simulink model "sensorMCUSlugsMKII_greg"  (Simulink 6.6)
settings: Solver=FixedStepDiscrete  StartTime=0.0  StopTime=10.0  FixedStep=0.01  RelTol=1e-3
InitFcn:
  | mcuInit
values from neighbouring files (symbols this model uses):
  T = 0.01    [initGPS.m]    (also in mcuInit.m)
undefined symbols (not defined in the file or in its folder): baroMeanTemp, baroOffset, baroScale, baroTempK, baseHeight, baseTemp, cubeAccelGain, cubeGyroGain, gaind, getCubeData, getGpsMainData, getMag, hil_getEuler, hil_getRates, hil_getRawRead, hil_getVned, hil_getXYZ, hilRead, ISA_rho0, lapseRate, logData, magMeanTemp, magOffset, magScale, magTempK, pitMeanTemp, pitotOffset, pitotScale, pitTempK, polesd, powerOffset, powerScale, protParseDecode, sensorMCUInit, spiSend, tempOffset, tempScale, u1, u2, updateAirData, updateAttitude, updateBias, updateDiagnosticFl, updateDiagnosticSh, updateLoadData, updatePilotConsole, updatePosition, updateRawADCData, updateTimeStamp, y1, zerosd
libraries: dsPICdrivers x36, simulink x3, aerolibconvert2 x1
(part 2 of 2)

== system sensorMCUSlugsMKII_greg/Sensor Data/Sensor Suite/Low Pass Filtering,Temperature Compensation and Calibration/3D Filter ==
  In1 : Inport
  Demux : Demux  Outputs=3
  Filter1 : Subsystem  mask(DiscretizedZeroPole){Zeros=zval, Poles=pval, Gain=kval, AbsTol=auto, SampleTime=TSample, method=tustin, Wc=1}
      mask prompts: Zeros "Zeros (enter in s-main:)"; Poles "Poles (enter in s-domain:)"; Gain "Gain (enter in s-domain:)"; AbsTol "Absolute tolerance:"; SampleTime "Sample time:"; Wc "Critical Frequency (Hz):"
      mask help: Continuous mask uses c2d to transform parameters onto the Discrete Zero-Pole block inside.
      mask init: same as sensorMCUSlugsMKII_greg/Sensor Data/Sensor Suite/Low Pass Filtering,Temperature Compensation and Calibration/Low Pass1
      mask StyleString: edit,edit,edit,edit,edit,popup(zoh|foh|tustin|prewarp|matched),edit
      mask CallbackString: |||||hidecrit|
      mask Display:
      | droots(zeross,poless,gainss)
      | text( 0.5, 1.0, method, 'verticalAlignment','top')
  Filter2 : Subsystem  mask(DiscretizedZeroPole){Zeros=zval, Poles=pval, Gain=kval, AbsTol=auto, SampleTime=TSample, method=tustin, Wc=1}
      mask prompts: Zeros "Zeros (enter in s-main:)"; Poles "Poles (enter in s-domain:)"; Gain "Gain (enter in s-domain:)"; AbsTol "Absolute tolerance:"; SampleTime "Sample time:"; Wc "Critical Frequency (Hz):"
      mask help: Continuous mask uses c2d to transform parameters onto the Discrete Zero-Pole block inside.
      mask init: same as sensorMCUSlugsMKII_greg/Sensor Data/Sensor Suite/Low Pass Filtering,Temperature Compensation and Calibration/Low Pass1
      mask StyleString: edit,edit,edit,edit,edit,popup(zoh|foh|tustin|prewarp|matched),edit
      mask CallbackString: |||||hidecrit|
      mask Display:
      | droots(zeross,poless,gainss)
      | text( 0.5, 1.0, method, 'verticalAlignment','top')
  Filter3 : Subsystem  mask(DiscretizedZeroPole){Zeros=zval, Poles=pval, Gain=kval, AbsTol=auto, SampleTime=TSample, method=tustin, Wc=1}
      mask prompts: Zeros "Zeros (enter in s-main:)"; Poles "Poles (enter in s-domain:)"; Gain "Gain (enter in s-domain:)"; AbsTol "Absolute tolerance:"; SampleTime "Sample time:"; Wc "Critical Frequency (Hz):"
      mask help: Continuous mask uses c2d to transform parameters onto the Discrete Zero-Pole block inside.
      mask init: same as sensorMCUSlugsMKII_greg/Sensor Data/Sensor Suite/Low Pass Filtering,Temperature Compensation and Calibration/Low Pass1
      mask StyleString: edit,edit,edit,edit,edit,popup(zoh|foh|tustin|prewarp|matched),edit
      mask CallbackString: |||||hidecrit|
      mask Display:
      | droots(zeross,poless,gainss)
      | text( 0.5, 1.0, method, 'verticalAlignment','top')
  myMux Fun1 : Stateflow chart
  Out1 : Outport
  wires:
  myMux Fun1/1(y) -> Out1/1
  In1/1 -> Demux/1
  Filter3/1(Out1) -> myMux Fun1/3(u3)
  Filter2/1(Out1) -> myMux Fun1/2(u2)
  Filter1/1(Out1) -> myMux Fun1/1(u1)
  Demux/3 -> Filter3/1(In1)
  Demux/2 -> Filter2/1(In1)
  Demux/1 -> Filter1/1(In1)

== system sensorMCUSlugsMKII_greg/Sensor Data/Sensor Suite/Low Pass Filtering,Temperature Compensation and Calibration/Baro Altimeter ==
  Static (Pa) : Inport  Orientation=up
  Compute Barometric Height : Subsystem  mask{baseTemp=baseTemp, LapseRate=lapseRate}
      mask prompts: baseTemp "Base Station Temperature (K)"; LapseRate "Lapse Rate (C/ft)"
      mask help:
      | Produces Altitude in meters from Barometric Pressure in Pascals. Altitude is valid from MSL to 6000 ft.
      |
      | The method implemented here was developed by Ren Curry
  Constant1 : Constant  Value=baseHeight  OutDataTypeMode=single
  Enabled Subsystem : Subsystem  TreatAsAtomicUnit=on
  Enables/Disables the Computation of  initial Baro Bias : Stateflow chart
  Initial Baro Bias : Subsystem  TreatAsAtomicUnit=on
  Logical Operator : Logic  Orientation=down  Operator=NOT  AllPortsSameDT=off  OutDataTypeMode=Boolean
  Sum1 : Sum  Inputs=++|  OutDataTypeMode=single
  Zero Out Height : Subsystem  TreatAsAtomicUnit=on
  Altitude : Outport
  wires:
  Compute Barometric Height/1("Altitude, m") -> Zero Out Height/2(Computed Height), Sum1/2
  Static (Pa)/1 -> Initial Baro Bias/1(Baro (Pa)), Compute Barometric Height/3(Baro (Pa))
  Enables/Disables the Computation of  initial Baro Bias/1(tOut) -> Initial Baro Bias/Enable, Zero Out Height/Enable, Logical Operator/1
  Constant1/1 -> Compute Barometric Height/1(Base Height (m)), Zero Out Height/1(Base Height)
  Initial Baro Bias/1(Baro (Gnd)) -> Compute Barometric Height/2(Base Pressure (Pa))
  Zero Out Height/1(Height Offset) -> Sum1/1
  Logical Operator/1 -> Enabled Subsystem/Enable
  Sum1/1 -> Enabled Subsystem/1(In1)
  Enabled Subsystem/1(Out1) -> Altitude/1

== system sensorMCUSlugsMKII_greg/Sensor Data/Sensor Suite/Low Pass Filtering,Temperature Compensation and Calibration/Baro Temp Compensation ==
  Raw : Inport
  Temp Raw : Inport  Port=2
  Divide1 : Product  OutDataTypeMode=single  OutScaling=2^-10
  Mean Temperature for Calibration : Constant  Value=tempMean  OutDataTypeMode=single
  Sum1 : Sum  Inputs=|+-  OutDataTypeMode=single
  Sum2 : Sum  Inputs=|+-  OutDataTypeMode=single
  gains : Constant  Value=alpha  OutDataTypeMode=single
  Comp : Outport
  wires:
  Mean Temperature for Calibration/1 -> Sum1/2
  Raw/1 -> Sum2/1
  Temp Raw/1 -> Sum1/1
  Sum1/1 -> Divide1/2
  gains/1 -> Divide1/1
  Divide1/1 -> Sum2/2
  Sum2/1 -> Comp/1

== system sensorMCUSlugsMKII_greg/Sensor Data/Sensor Suite/Low Pass Filtering,Temperature Compensation and Calibration/Barometer Unit Conversion ==
  Raw : Inport
  Bias : Constant  Value=bias  OutDataTypeMode=single
  Divide : Product  OutDataTypeMode=single  OutScaling=2^-10
  Gains : Constant  Value=gains  OutDataTypeMode=single
  Sum : Sum  Inputs=|++  OutDataTypeMode=single
  Comp : Outport
  wires:
  Bias/1 -> Sum/2
  Raw/1 -> Divide/2
  Gains/1 -> Divide/1
  Divide/1 -> Sum/1
  Sum/1 -> Comp/1

== system sensorMCUSlugsMKII_greg/Sensor Data/Sensor Suite/Low Pass Filtering,Temperature Compensation and Calibration/Low Pass1 ==
  In1 : Inport
  Discrete Zero-Pole : DiscreteZeroPole  Zeros=zerosd  Poles=polesd  Gain=gaind  SampleTime=SampleTime
  Out1 : Outport
  wires:
  In1/1 -> Discrete Zero-Pole/1
  Discrete Zero-Pole/1 -> Out1/1

== system sensorMCUSlugsMKII_greg/Sensor Data/Sensor Suite/Low Pass Filtering,Temperature Compensation and Calibration/Low Pass2 ==
  In1 : Inport
  Discrete Zero-Pole : DiscreteZeroPole  Zeros=zerosd  Poles=polesd  Gain=gaind  SampleTime=SampleTime
  Out1 : Outport
  wires:
  Discrete Zero-Pole/1 -> Out1/1
  In1/1 -> Discrete Zero-Pole/1

== system sensorMCUSlugsMKII_greg/Sensor Data/Sensor Suite/Low Pass Filtering,Temperature Compensation and Calibration/Low Pass4 ==
  In1 : Inport
  Discrete Zero-Pole : DiscreteZeroPole  Zeros=zerosd  Poles=polesd  Gain=gaind  SampleTime=SampleTime
  Out1 : Outport
  wires:
  Discrete Zero-Pole/1 -> Out1/1
  In1/1 -> Discrete Zero-Pole/1

== system sensorMCUSlugsMKII_greg/Sensor Data/Sensor Suite/Low Pass Filtering,Temperature Compensation and Calibration/Low Pass8 ==
  In1 : Inport
  Discrete Zero-Pole : DiscreteZeroPole  Zeros=zerosd  Poles=polesd  Gain=gaind  SampleTime=SampleTime
  Out1 : Outport
  wires:
  In1/1 -> Discrete Zero-Pole/1
  Discrete Zero-Pole/1 -> Out1/1

== system sensorMCUSlugsMKII_greg/Sensor Data/Sensor Suite/Low Pass Filtering,Temperature Compensation and Calibration/Magnetometer Unit Conversion ==
  Raw : Inport
  Bias : Constant  Value=bias  OutDataTypeMode=single
  Divide : Product  OutDataTypeMode=single  OutScaling=2^-10
  Gains : Constant  Value=gains  OutDataTypeMode=single
  Sum : Sum  Inputs=|++  OutDataTypeMode=single
  Comp : Outport
  wires:
  Sum/1 -> Comp/1
  Divide/1 -> Sum/1
  Gains/1 -> Divide/1
  Raw/1 -> Divide/2
  Bias/1 -> Sum/2

== system sensorMCUSlugsMKII_greg/Sensor Data/Sensor Suite/Low Pass Filtering,Temperature Compensation and Calibration/Magnetometers Temp Compensation ==
  Raw : Inport
  Temp Raw : Inport  Port=2
  Divide1 : Product  OutDataTypeMode=single  OutScaling=2^-10
  Mean Temperature for Calibration : Constant  Value=tempMean  OutDataTypeMode=single
  Sum1 : Sum  Inputs=|+-  OutDataTypeMode=single
  Sum2 : Sum  Inputs=|+-  OutDataTypeMode=single
  gains : Constant  Value=alpha  OutDataTypeMode=single
  Comp : Outport
  wires:
  Sum2/1 -> Comp/1
  Divide1/1 -> Sum2/2
  gains/1 -> Divide1/1
  Sum1/1 -> Divide1/2
  Temp Raw/1 -> Sum1/1
  Raw/1 -> Sum2/1
  Mean Temperature for Calibration/1 -> Sum1/2

== system sensorMCUSlugsMKII_greg/Sensor Data/Sensor Suite/Low Pass Filtering,Temperature Compensation and Calibration/Pitot Unit Conversion ==
  Raw : Inport
  Bias : Constant  Value=bias  OutDataTypeMode=single
  Divide : Product  OutDataTypeMode=single  OutScaling=2^-10
  Gains : Constant  Value=gains  OutDataTypeMode=single
  Sum : Sum  Inputs=|++  OutDataTypeMode=single
  Comp : Outport
  wires:
  Bias/1 -> Sum/2
  Raw/1 -> Divide/2
  Gains/1 -> Divide/1
  Divide/1 -> Sum/1
  Sum/1 -> Comp/1

== system sensorMCUSlugsMKII_greg/Sensor Data/Sensor Suite/Low Pass Filtering,Temperature Compensation and Calibration/Pitot Temp Compensation ==
  Raw : Inport
  Temp Raw : Inport  Port=2
  Divide1 : Product  OutDataTypeMode=single  OutScaling=2^-10
  Mean Temperature for Calibration : Constant  Value=tempMean  OutDataTypeMode=single
  Sum1 : Sum  Inputs=|+-  OutDataTypeMode=single
  Sum2 : Sum  Inputs=|+-  OutDataTypeMode=single
  gains : Constant  Value=alpha  OutDataTypeMode=single
  Comp : Outport
  wires:
  Mean Temperature for Calibration/1 -> Sum1/2
  Raw/1 -> Sum2/1
  Temp Raw/1 -> Sum1/1
  Sum1/1 -> Divide1/2
  gains/1 -> Divide1/1
  Divide1/1 -> Sum2/2
  Sum2/1 -> Comp/1

== system sensorMCUSlugsMKII_greg/Sensor Data/Sensor Suite/Low Pass Filtering,Temperature Compensation and Calibration/Power Unit Conversion ==
  Raw : Inport
  Bias : Constant  Value=bias  OutDataTypeMode=single
  Divide : Product  OutDataTypeMode=single  OutScaling=2^-10
  Gains : Constant  Value=gains  OutDataTypeMode=single
  Sum : Sum  Inputs=|++  OutDataTypeMode=single
  Comp : Outport
  wires:
  Bias/1 -> Sum/2
  Raw/1 -> Divide/2
  Gains/1 -> Divide/1
  Divide/1 -> Sum/1
  Sum/1 -> Comp/1

== system sensorMCUSlugsMKII_greg/Sensor Data/Sensor Suite/Low Pass Filtering,Temperature Compensation and Calibration/Thermistor Unit Conversion ==
  Raw : Inport
  Bias : Constant  Value=bias  OutDataTypeMode=single
  Divide : Product  OutDataTypeMode=single  OutScaling=2^-10
  Gains : Constant  Value=gains  OutDataTypeMode=single
  Sum : Sum  Inputs=|++  OutDataTypeMode=single
  Comp : Outport
  wires:
  Sum/1 -> Comp/1
  Divide/1 -> Sum/1
  Gains/1 -> Divide/1
  Raw/1 -> Divide/2
  Bias/1 -> Sum/2

== system sensorMCUSlugsMKII_greg/Position-Attitude Filter/Position Filter/Geod2LTP2/ECEF2LTP (UEN)/From Body to Universal1 ==
  long : Inport
  lat : Inport  Port=2
  Mux : Mux  Inputs=2
  Reshape 9x1->3x1 : S-Function  FunctionName=sreshape  Parameters=OutputDimensionality, OutputDimensions  mask(Reshape){OutputDimensionality=Customize, OutputDimensions=[3,3]}
      mask prompts: OutputDimensionality "Output dimensionality:"; OutputDimensions "Output dimensions:"
      mask help:
      | Change the dimensions of a vector or matrix input signal. Output
      |  - a one-dimensional array (vector),
      |  - a column vector (Mx1 matrix),
      |  - a row vector (1xN matrix), or
      |  - a matrix or vector with specified dimensions, e.g., [M, N] or [W].
      mask init:
      | s = reshapemask(gcb,'init');
      mask StyleString: popup(1-D array|Column vector|Row vector|Customize),edit
      mask CallbackString: reshapemask(gcb,'cbDimensionality')|
      mask Display: disp('Reshape')
  Rotation Matrix from Long//Lat : Subsystem
      mask Type: Vector Transformation
      mask Description: Vector Transformation
      mask Display: disp('axis')
  DCM : Outport
  wires:
  lat/1 -> Mux/2
  long/1 -> Mux/1
  Mux/1 -> Rotation Matrix from Long//Lat/1(long lat)
  Rotation Matrix from Long//Lat/1(DCM) -> Reshape 9x1->3x1/1
  Reshape 9x1->3x1/1 -> DCM/1

== system sensorMCUSlugsMKII_greg/Position-Attitude Filter/Position Filter/Geod2LTP2/Geod2ECEF/eccentricity^2 ==
  " " : Product  SaturateOnIntegerOverflow=on  InputSameDT=on
  Re=equatorial radius1 : Constant  Value=Re
  Rp=polar radius : Constant  Value=Rp
  Sum5 : Sum  Inputs=|+-  SaturateOnIntegerOverflow=on  InputSameDT=on
  const2 : Constant
  e^1 : Product  Inputs=*/  SaturateOnIntegerOverflow=on  InputSameDT=on
  e^2 : Outport
  wires:
  Re=equatorial radius1/1 -> e^1/2
  Rp=polar radius/1 -> e^1/1
  const2/1 -> Sum5/1
  e^1/1 -> " "/2, " "/1
  " "/1 -> Sum5/2
  Sum5/1 -> e^2/1

== system sensorMCUSlugsMKII_greg/Position-Attitude Filter/Position Filter/Geod2LTP2/Geod2ECEF1/eccentricity^2 ==
  " " : Product  SaturateOnIntegerOverflow=on  InputSameDT=on
  Re=equatorial radius1 : Constant  Value=Re
  Rp=polar radius : Constant  Value=Rp
  Sum5 : Sum  Inputs=|+-  SaturateOnIntegerOverflow=on  InputSameDT=on
  const2 : Constant
  e^1 : Product  Inputs=*/  SaturateOnIntegerOverflow=on  InputSameDT=on
  e^2 : Outport
  wires:
  Sum5/1 -> e^2/1
  " "/1 -> Sum5/2
  e^1/1 -> " "/1, " "/2
  const2/1 -> Sum5/1
  Rp=polar radius/1 -> e^1/1
  Re=equatorial radius1/1 -> e^1/2

== system sensorMCUSlugsMKII_greg/Sensor Data/Sensor Suite/Low Pass Filtering,Temperature Compensation and Calibration/3D Filter/Filter1 ==
  In1 : Inport
  Discrete Zero-Pole : DiscreteZeroPole  Zeros=zerosd  Poles=polesd  Gain=gaind  SampleTime=SampleTime
  Out1 : Outport
  wires:
  Discrete Zero-Pole/1 -> Out1/1
  In1/1 -> Discrete Zero-Pole/1

== system sensorMCUSlugsMKII_greg/Sensor Data/Sensor Suite/Low Pass Filtering,Temperature Compensation and Calibration/3D Filter/Filter2 ==
  In1 : Inport
  Discrete Zero-Pole : DiscreteZeroPole  Zeros=zerosd  Poles=polesd  Gain=gaind  SampleTime=SampleTime
  Out1 : Outport
  wires:
  In1/1 -> Discrete Zero-Pole/1
  Discrete Zero-Pole/1 -> Out1/1

== system sensorMCUSlugsMKII_greg/Sensor Data/Sensor Suite/Low Pass Filtering,Temperature Compensation and Calibration/3D Filter/Filter3 ==
  In1 : Inport
  Discrete Zero-Pole : DiscreteZeroPole  Zeros=zerosd  Poles=polesd  Gain=gaind  SampleTime=SampleTime
  Out1 : Outport
  wires:
  Discrete Zero-Pole/1 -> Out1/1
  In1/1 -> Discrete Zero-Pole/1

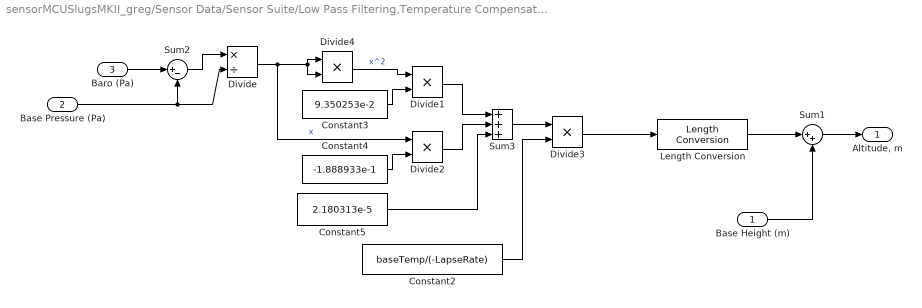
== system sensorMCUSlugsMKII_greg/Sensor Data/Sensor Suite/Low Pass Filtering,Temperature Compensation and Calibration/Baro Altimeter/Compute Barometric Height ==
  Base Height (m) : Inport
  Base Pressure (Pa) : Inport  Port=2
  Baro (Pa) : Inport  Port=3
  Constant2 : Constant  Value=baseTemp/(-LapseRate)  OutDataTypeMode=single
  Constant3 : Constant  Value=9.350253e-2  OutDataTypeMode=single
  Constant4 : Constant  Value=-1.888933e-1  OutDataTypeMode=single
  Constant5 : Constant  Value=2.180313e-5  OutDataTypeMode=single
  Divide : Product  Inputs=*/  OutDataTypeMode=single  OutScaling=2^-10
  Divide{1..4} (4 alike) : Product  OutDataTypeMode=single  OutScaling=2^-10
  Length Conversion : aerolibconvert2/Length Conversion  SystemSampleTime=-1  IU=ft  OU=m
  Sum1 : Sum  Inputs=|++  OutDataTypeMode=single
  Sum2 : Sum  Inputs=|+-  OutDataTypeMode=single
  Sum3 : Sum  Inputs=3  OutDataTypeMode=single
  "Altitude, m" : Outport
  wires:
  Length Conversion/1 -> Sum1/1
  Sum2/1 -> Divide/1
  Sum1/1 -> "Altitude, m"/1
  Divide3/1 -> Length Conversion/1
  Constant2/1 -> Divide3/2
  Sum3/1 -> Divide3/1
  Constant5/1 -> Sum3/3
  Divide2/1 -> Sum3/2
  Divide1/1 -> Sum3/1
  Constant4/1 -> Divide2/2
  Constant3/1 -> Divide1/2
  Divide4/1 -> Divide1/1  "x^2"
  Divide/1 -> Divide2/1, Divide4/1, Divide4/2  "x"
  Base Pressure (Pa)/1 -> Divide/2, Sum2/2
  Base Height (m)/1 -> Sum1/2
  Baro (Pa)/1 -> Sum2/1

== system sensorMCUSlugsMKII_greg/Sensor Data/Sensor Suite/Low Pass Filtering,Temperature Compensation and Calibration/Baro Altimeter/Enabled Subsystem ==
  In1 : Inport
  Enable : EnablePort
  Out1 : Outport  InitialOutput=baseHeight
  wires:
  In1/1 -> Out1/1

== system sensorMCUSlugsMKII_greg/Sensor Data/Sensor Suite/Low Pass Filtering,Temperature Compensation and Calibration/Baro Altimeter/Initial Baro Bias ==
  Baro (Pa) : Inport
  Enable : EnablePort
  Data Type Conversion : DataTypeConversion  OutDataTypeMode=double
  Data Type Conversion1 : DataTypeConversion  OutDataTypeMode=single
  Low Pass8 : Subsystem  mask(DiscretizedZeroPole){Zeros=[], Poles=[-3], Gain=3, AbsTol=auto, SampleTime=.01, method=tustin, Wc=1}
      mask prompts: Zeros "Zeros (enter in s-main:)"; Poles "Poles (enter in s-domain:)"; Gain "Gain (enter in s-domain:)"; AbsTol "Absolute tolerance:"; SampleTime "Sample time:"; Wc "Critical Frequency (Hz):"
      mask help: Continuous mask uses c2d to transform parameters onto the Discrete Zero-Pole block inside.
      mask init: same as sensorMCUSlugsMKII_greg/Sensor Data/Sensor Suite/Low Pass Filtering,Temperature Compensation and Calibration/Low Pass1
      mask StyleString: edit,edit,edit,edit,edit,popup(zoh|foh|tustin|prewarp|matched),edit
      mask CallbackString: |||||hidecrit|
      mask Display:
      | droots(zeross,poless,gainss)
      | text( 0.5, 1.0, method, 'verticalAlignment','top')
  Mux : Mux  Inputs=2
  Scope : Scope
      settings: SaveName=ScopeData8
  "[80k - 120k]" : Saturate  UpperLimit=120000  LowerLimit=80000
  Baro (Gnd) : Outport
  wires:
  Baro (Pa)/1 -> Data Type Conversion/1
  Low Pass8/1(Out1) -> Data Type Conversion1/1
  Data Type Conversion/1 -> Low Pass8/1(In1)
  Data Type Conversion1/1 -> Mux/2, "[80k - 120k]"/1
  Mux/1 -> Scope/1
  "[80k - 120k]"/1 -> Baro (Gnd)/1, Mux/1

== system sensorMCUSlugsMKII_greg/Sensor Data/Sensor Suite/Low Pass Filtering,Temperature Compensation and Calibration/Baro Altimeter/Zero Out Height ==
  Base Height : Inport
  Computed Height : Inport  Port=2
  Enable : EnablePort
  Integer Delay : simulink/Discrete/Integer Delay  vinit=0  samptime=.01  NumDelays=1
  Sum : Sum  Inputs=|+-  OutDataTypeMode=single
  Height Offset : Outport
  wires:
  Computed Height/1 -> Integer Delay/1
  Sum/1 -> Height Offset/1
  Integer Delay/1 -> Sum/2
  Base Height/1 -> Sum/1

== system sensorMCUSlugsMKII_greg/Position-Attitude Filter/Position Filter/Geod2LTP2/ECEF2LTP (UEN)/From Body to Universal1/Rotation Matrix from Long//Lat ==
  note: Calculate Coefficients of DCM Row-Wise
  long lat : Inport
  11 : Fcn  Expr=cos(u[1])*cos(u[2])
  12 : Fcn  Expr=sin(u[1])*cos(u[2])
  13 : Fcn  Expr=sin(u[2])
  21 : Fcn  Expr=-sin(u[1])
  22 : Fcn  Expr=cos(u[1])
  23 : Fcn  Expr=0
  31 : Fcn  Expr=-sin(u[2])*cos(u[1])
  32 : Fcn  Expr=-sin(u[1])*sin(u[2])
  33 : Fcn  Expr=cos(u[2])
  Mux2 : Mux  Inputs=9
  DCM : Outport  InitialOutput=0
  wires:
  33/1 -> Mux2/9
  23/1 -> Mux2/8
  13/1 -> Mux2/7
  32/1 -> Mux2/6
  22/1 -> Mux2/5
  12/1 -> Mux2/4
  31/1 -> Mux2/3
  21/1 -> Mux2/2
  11/1 -> Mux2/1
  Mux2/1 -> DCM/1
  long lat/1 -> 11/1, 33/1, 23/1, 13/1, 32/1, 22/1, 12/1, 31/1, 21/1

== system sensorMCUSlugsMKII_greg/Sensor Data/Sensor Suite/Low Pass Filtering,Temperature Compensation and Calibration/Baro Altimeter/Initial Baro Bias/Low Pass8 ==
  In1 : Inport
  Discrete Zero-Pole : DiscreteZeroPole  Zeros=zerosd  Poles=polesd  Gain=gaind  SampleTime=SampleTime
  Out1 : Outport
  wires:
  In1/1 -> Discrete Zero-Pole/1
  Discrete Zero-Pole/1 -> Out1/1

== matlab function Sensor Data/Sensor Suite/myMux Fun ==
  data: u1 input inherited; y output inherited; u2 input inherited; u3 input inherited
function y = myMux3(u1, u2, u3)
% This block supports an embeddable subset of the MATLAB language.
% See the help menu for details. 

y = [u1(1); u2(1); u3(1)];

== matlab function myMux Fun1 ==
  data: u1 input inherited; y output inherited; u2 input inherited; u3 input inherited
function y = myMux3(u1, u2, u3)
% This block supports an embeddable subset of the MATLAB language.
% See the help menu for details. 

y = [u1(1); u2(1); u3(1)];

== matlab function myMux Fun5 ==
  data: u1 input inherited; y output inherited; u2 input inherited; u3 input inherited
function y = myMux3(u1, u2, u3)
% This block supports an embeddable subset of the MATLAB language.
% See the help menu for details. 

y = [u1(1); u2(1); u3(1)];

== matlab function myMux Fun4 ==
  data: u1 input inherited; y output inherited; u2 input inherited
function y = myMux(u1, u2)
% This block supports an embeddable subset of the MATLAB language.
% See the help menu for details. 

y = [u1(1:3); u2(1:3)];

== matlab function myMux Fun3 ==
  data: u1 input inherited; y output inherited; u2 input inherited
function y = myMux(u1, u2)
% This block supports an embeddable subset of the MATLAB language.
% See the help menu for details. 

y = [u1(1:3); u2(1:3)];

== matlab function Sensor Data/Sensor Suite/Low Pass Filtering,Temperature Compensation and Calibration/3D Filter/myMux Fun1 ==
  data: u1 input inherited; y output inherited; u2 input inherited; u3 input inherited
function y = myMux(u1, u2, u3)
% This block supports an embeddable subset of the MATLAB language.
% See the help menu for details. 

y = [u1(1); u2(1); u3(1)];

== matlab function Sensor Data/Sensor Suite/Low Pass Filtering,Temperature Compensation and Calibration/Baro Altimeter/Enables/Disables the Computation of initial Baro Bias ==
  data: tOut output inherited
function tOut = getTIni

persistent aveCount;
persistent tIni;

if isempty(aveCount)
    aveCount =1;
    tIni = 1;
end;

if aveCount < 2500
    aveCount = aveCount + 1;
end

if aveCount == 2500
    tIni =0;
    aveCount = aveCount + 1;
end

tOut = tIni;

%if aveCount > 500
%    tIni = 0;
%end

% if isempty(aveCount)
%     aveCount =1;
%     initBias = [0.0 0.0 0.0]';
% end;
%     
% if (aveCount<10)
%     initBias = initBias+ Raw;
%     bias = initBias/aveCount;
%     aveCount = aveCount +1;
% end;
% 
% if (aveCount == 10)
%     initBias = initBias/(aveCount-1);
%     aveCount = 100;
% end;
% 
% if (aveCount == 100)
%     bias = initBias;
% end;

== matlab function Position-Attitude Filter/Position Filter/GPS2LLH ==
  data: GPS input inherited; LLH output inherited
function LLH  = fcn(GPS)
% This block supports an embeddable subset of the MATLAB language.
% See the help menu for details. 

LLH=GPS(1:3);

== matlab function Position-Attitude Filter/EKF ==
  data: quatout output single; bias_out output single; V_inertial_out output single; gyros input single; accels input single; mags input single; XYZ_inertial input single; gps_update input single; dt_gps input single; euler_out output single; pqr_out output single; unfiltered_euler_out output single; bodyAcc_out output single; P_out output single
function [quatout,bias_out,V_inertial_out,euler_out,pqr_out,unfiltered_euler_out,bodyAcc_out,P_out] = fcn(gyros,accels,mags,XYZ_inertial,gps_update,dt_gps)

    %%************************************************************
    %%***************** initialize variables *********************
    %%************************************************************
    persistent xhat;
    persistent P;
	persistent XYZ_inertial_prev;
    persistent XYZ_inertial_prev_prev;
    persistent unfiltered_euler;
    persistent bodyAcc;
    persistent V_inertial;
    persistent gyros_old;

    if isempty(xhat)
%         xhat = [0.4;
%                  -.15;
%                  .2;
%                -0.9;
%                 [0;0;0]];
% %        P=diag( [1^2*ones(1,3) .1^2*ones(1,3) ] );
%         P=diag( [.1^2*ones(1,3) .01^2*ones(1,3)] );
%         XYZ_inertial_prev = [0;0;0];
%         XYZ_inertial_prev_prev = [0;0;0];        
%         unfiltered_euler = [0;0;0];
%         bodyAcc = [0;0;0];
%         V_inertial = [0;0;0];
%         gps_alive = 0;
%         gyros_old = gyros;
        xhat = single([0.4;
                 -.15;
                 .2;
               -0.9;
                1e-6.*[1;1;1]]);
%        P=diag( [1^2*ones(1,3) .1^2*ones(1,3) ] );
        P=single(diag( [1^2*ones(1,3) .001^2*ones(1,3)] ));
        XYZ_inertial_prev = single([0;0;0]);
        XYZ_inertial_prev_prev = single([0;0;0]);        
        unfiltered_euler = single([0;0;0]);
        bodyAcc = single([0;0;0]);
        V_inertial = single([0;0;0]);
        gps_alive = 0;
        gyros_old = gyros;
    
    end

    dt = single(0.01); % fundamental time step
    g  = single(9.81);
    B=single([23134.;
              5832.5;
              42481.;]); %magnetic field NED in nanoteslas, June 11 2009, Santa Cruz
    B=B/norm(B); %normalize magnetic field

%     a_n = single(4);
%     m_n = single(.05);
    a_n = single(50);
    m_n = single(.6);  
%     a_n = 4e2;
%     m_n = .05e2;
    Q_quat = single(1e-5);
%	Q_quat = single(1e-4);
 %   Q_bias = single(0.00128); % discreet noise (100Hz) in radians/sec
    Q_bias = single(1e-2);
   tau_gyro = single(100);
%   tau_gyro = single(500);
   exptau =single(exp(-dt/tau_gyro));    

%    R = diag(q_n^2*ones(1,3));
    R_sens = diag([a_n^2*ones(1,3) m_n^2*ones(1,3)]);
    Q = diag([Q_quat^2*ones(1,3) dt*Q_bias^2*ones(1,3)]);

    x_old=xhat;
    
    %%************************************************************
    %%******************** propogate state ***********************
    %%************************************************************
    p  = gyros_old(1)-x_old(5);
    q  = gyros_old(2)-x_old(6);
    r  = gyros_old(3)-x_old(7);
    
    normomega    = single(norm([p;q;r]));
    normomegainv = inv(normomega);
    C  = cos(.5*dt*normomega);
    Sn = sin(.5*dt*normomega)*normomegainv;

    Phi_old_small = [    C, -(p *Sn), -(q* Sn), -(r *Sn);
                   (p *Sn),        C,  (r* Sn), -(q *Sn);
                   (q* Sn), -(r *Sn),        C,  (p* Sn);
                   (r* Sn),  (q *Sn), -(p* Sn),        C;];
    x_minus=[Phi_old_small*x_old(1:4);     %(predict state)
                          x_old(5:7);];
    if x_minus(1)<0
        x_minus(1:4)=-x_minus(1:4);
    end
    x_minus(1:4) = x_minus(1:4)/norm(x_minus(1:4));  %normalize quaternion



	%%*************************************************************
    %%************ propogate covariance ***************************
    %%*************************************************************
    %old state transition matrix
%     Phi_old = [1,0,0,-.5*dt,     0,     0;
%                0,1,0,     0,-.5*dt,     0;
%                0,0,1,     0,     0,-.5*dt;
%                0,0,0,     1,     0,     0;
%                0,0,0,     0,     1,     0;
%                0,0,0,     0,     0,     1;];
           
    Phi_old = single([1,0,0,-.5*dt,     0,     0;
                      0,1,0,     0,-.5*dt,     0;
                      0,0,1,     0,     0,-.5*dt;
                      0,0,0,exptau,     0,     0;
                      0,0,0,     0,exptau,     0;
                      0,0,0,     0,     0,exptau;]);
           
    % propogate covariance
%     P = Phi_old*(P+Q)*transpose(Phi_old); %too slow
    P = [P(1:3,1:3)+Q(1:3,1:3)+.5*dt*( -transpose(P(1:3,4:6)) - P(1:3,4:6) + .5*dt*(P(4:6,4:6)+Q(4:6,4:6)) ), exptau*(P(1:3,4:6)-.5*dt*(P(4:6,4:6)+Q(4:6,4:6)));
         zeros(3,3), exptau^2*(P(4:6,4:6)+Q(4:6,4:6))];  %this is faster
    P(4:6,1:3)=transpose(P(1:3,4:6));                    %this is faster 

    %% ***********************************************************************
    %% ******** translational filter *****************************************
    %% ***********************************************************************
    %% check for gps update
    if gps_update
        V_inertial = (XYZ_inertial-XYZ_inertial_prev)/dt_gps;
        Cnb = q2dcm(x_minus(1:4));
    
        bodyAcc = Cnb*((XYZ_inertial-2*XYZ_inertial_prev+XYZ_inertial_prev_prev)/(dt_gps^2));
        if ((XYZ_inertial_prev_prev(1) == 0) && (XYZ_inertial_prev_prev(2) == 0))
            bodyAcc = single([0;0;0]);
        end
        XYZ_inertial_prev_prev = XYZ_inertial_prev;
        XYZ_inertial_prev=XYZ_inertial;

    
    %% ***********************************************************************
    %% ********************* update ******************************************
    %% ***********************************************************************
        qm = xhat(1:4);
        MM= single(zeros(3,6));
        M = single(zeros(6,3));
        W = single(zeros(6,6));
    
        Cnb = q2dcm(qm);
        A_hat = Cnb*[0;0;-g];
        B_hat = Cnb*B;
        M = [2*sk(A_hat);2*sk(B_hat)]; %no noise
%        M = [2*sk(A_hat)./a_n;2*sk(B_hat)./m_n]; %include noise
        W = diag([1/a_n^2*[1 1 1] 1/m_n^2*[1 1 1]]);
%        MM = inv(transpose(M)*M)*transpose(M); %no noise
        MM = inv(transpose(M)*W*M)*transpose(M)*W; %with noise

        q__err = MM*[ ((accels-bodyAcc)-A_hat) ; (mags-B_hat) ]; %no noise
        %q__err = MM*[ ((accels-bodyAcc)-A_hat)./a_n ; (mags-B_hat)./m_n ]; %include noise

%             if norm(q__err)^2 < 1
%                 qm=quatmult([sqrt(1-norm(q__err)^2);q__err],qm);
%             else
%        qm=quatmult(qm,[1;q__err]);
        qm=quatmult(qm,[1;q__err]);
%            end
        if (qm(1)<0)
            qm = -qm;            					% make scalar part positive
        end
        qm=qm/norm(qm);
    
        unfiltered_euler=quat2eul(qm);
    
%    z_temp = quatmult(qm,quatinv(xhat(1:4)));
%    z=z_temp(2:4);
        z=q__err;
    % Expected measurement
        z_hat = [0;0;0];

    % Linearized measurement matrix H
        H= [eye(3,3) zeros(3,3)];
%    R= inv(transpose(M)*W*M); %with noise
   % R=diag(q_n^2*ones(1,3)); %no noise
        R=MM*R_sens*transpose(MM);
    
%     K = P*H'*inv(H*P*H'+R);	% kalman gain, too slow
    % this is faster:
        HinvHPHpR = [inv(P(1:3,1:3)+R);
                        zeros(3,3)];    
        K = [P(1:3,1:3)*HinvHPHpR(1:3,1:3);
            transpose(P(1:3,4:6))*HinvHPHpR(1:3,1:3)];

%     P = (eye(6)-K*H)*P; % update covariance, too slow
        P = [(eye(3)-K(1:3,1:3))*P(1:3,1:3), (eye(3)-K(1:3,1:3))*P(1:3,4:6);        %faster
            -K(4:6,1:3)*P(1:3,1:3)+transpose(P(1:3,4:6)), -K(4:6,1:3)*P(1:3,4:6)+P(4:6,4:6)];
        xerror_hat = [zeros(3,1);x_old(5:7)]+K*(z-z_hat); % update state
        xhat(5:7)=xerror_hat(4:6);
        xhat(1:4)=quatmult(x_minus(1:4),[1;xerror_hat(1:3)]);
    else
        xhat = x_minus;
        unfiltered_euler = single([0;0;0]);
    end


    if xhat(1)<0
        xhat(1:4)=-xhat(1:4);
    end
    xhat(1:4) = xhat(1:4)./norm(xhat(1:4)); %normalize quaternion

    gyros_old = gyros; %save for next time
    
    %% ***********************************************************************
    %% ********************* unfiltered euler angles *************************
    %% ***********************************************************************
%     Gbody = accels-bodyAcc;
%     Gbody = Gbody/norm(Gbody)*.99999999;
%     Pitch = asin(Gbody(1));
%     temp = -Gbody(2)/cos(Pitch);
%     if abs(temp)<1
%     	Roll = asin(-Gbody(2)/cos(Pitch));
%     else
%     	Roll = pi/2*sign(temp);
%     end
%         
% 	if sign(Gbody(3)) >= 0   % if upside down, correct phi
%         Roll=-Roll-pi*sign(Gbody(2));
% 	end
% 
%     ct = cos(Pitch); %set up trig for less computation time
%     st = sin(Pitch);
%     cp = cos(Roll);
%     sp = sin(Roll);
%     Bflat = [ct, st*sp, cp*st;
%               0,    cp,   -sp;]*mags; %rotate mags into phi=0, theta=0
% 	Yaw = 0.2686 -atan2g(Bflat(2),Bflat(1)); %calculate psi
%     unfiltered_euler = [Pitch;Roll;Yaw];

    
    %% ***********************************************************************
    %% ********************* outputs *****************************************
    %% ***********************************************************************
    P_out = P;
    quatout = xhat(1:4);
    euler_out = quat2eul(quatout);
%    euler_out(1) = -euler_out(1); %reverse sign for GS
    bias_out = xhat(5:7);
    pqr_out = gyros-xhat(5:7);

    unfiltered_euler_out = unfiltered_euler;
    bodyAcc_out = bodyAcc;
    V_inertial_out = V_inertial;
    
end














%================================================================
%==================   additional functions ======================
%================================================================
function quat = integ_gyros(xhat,w,dt)
    p  = w(1) - xhat(5);
    q  = w(2) - xhat(6);
    r  = w(3) - xhat(7);
    normomega    = norm([p;q;r]);
    normomegainv = inv(normomega);
    C  = cos(.5*dt*normomega);
    Sn = sin(.5*dt*normomega)*normomegainv;

    Phi_old_small = [    C, -(p *Sn), -(q* Sn), -(r *Sn);
                   (p *Sn),        C,  (r* Sn), -(q *Sn);
                   (q* Sn), -(r *Sn),        C,  (p* Sn);
                   (r* Sn),  (q *Sn), -(p* Sn),        C;];
    xhat(1:4) = Phi_old_small*xhat(1:4);	       % insert back into state
    if xhat(1)<0
        xhat(1:4)=-xhat(1:4);
    end
    quat = xhat(1:4)/norm(xhat(1:4));  %normalize quaternion
end


function [Pitch, Roll, Yaw] = accelMagsBody2euler(acc,mags,body)
    Gbody = acc-body;
    Gbody = Gbody/norm(Gbody)*.99999999;
    Pitch = asin(Gbody(1));
    temp = -Gbody(2)/cos(Pitch);
    if abs(temp)<1
    	Roll = asin(-Gbody(2)/cos(Pitch));
    else
    	Roll = pi/2*sign(temp);
    end
        
	if sign(Gbody(3)) >= 0   % if upside down, correct phi
        Roll=-Roll-pi*sign(Gbody(2));
	end

    ct = cos(Pitch); %set up trig for less computation time
    st = sin(Pitch);
    cp = cos(Roll);
    sp = sin(Roll);
    Bflat = [ct, st*sp, cp*st;
              0,    cp,   -sp;]*mags; %rotate mags into phi=0, theta=0
	Yaw = 0.2686 -atan2g(Bflat(2),Bflat(1)); %calculate psi
end


function as=sk(a)
    % This function determines the skew-symmetric matrix
    % corresponding to a given vector a with three elements.
    	as=[0 -a(3) a(2); a(3) 0 -a(1); -a(2) a(1) 0];
end


function quat = quatmult(q1,q2)
    %   Multiplies two quaternions.
    qv1 = q1(2:4);
    qs1 = q1(1);
    qv2 = q2(2:4);
    qs2 = q2(1);

    quatv = cross(qv1,qv2) + qs1*qv2 + qs2*qv1;
    quats = qs1*qs2 - dot(qv1,qv2);

    quat = [quats;quatv];
end


function quat = quatinv(q)
    %   Inverts a quaternion.
    quat = [q(1);-q(2:4)];
end


function angles = quat2eul( q )
    qin = q./norm(q);

    y=2.*(qin(3,1).*qin(4,1) + qin(1,1).*qin(2,1));
    x=qin(1,1).^2 - qin(2,1).^2 - qin(3,1).^2 + qin(4,1).^2;
    phi = atan2g(y,x);

    theta = asin(-2.*(qin(2,1).*qin(4,1) - qin(1,1).*qin(3,1)));

    y=2.*(qin(2,1).*qin(3,1) + qin(1,1).*qin(4,1));
    x=qin(1,1).^2 + qin(2,1).^2 - qin(3,1).^2 - qin(4,1).^2;
    psi = atan2g(y,x);

    angles = [phi; theta; psi];
end


function angle = atan2g(y,x)
    angle = single(0.);
    if x>0
        angle = atan(y/x);
    end
    if x==0
        angle = .5*pi*sign(y);
    end
    if x<0
        angle = pi*sign(y)+atan(y/x);
    end
end

function q = eul2quat(angles)
    % converts phi,theta,phi into q
    % lifted straight from matlab's function (with a transposed output):
    cang = cos( angles/2 );
    sang = sin( angles/2 );

    q = [ cang(:,1).*cang(:,2).*cang(:,3) + sang(:,1).*sang(:,2).*sang(:,3);
           sang(:,1).*cang(:,2).*cang(:,3) - cang(:,1).*sang(:,2).*sang(:,3);
           cang(:,1).*sang(:,2).*cang(:,3) + sang(:,1).*cang(:,2).*sang(:,3);
           cang(:,1).*cang(:,2).*sang(:,3) - sang(:,1).*sang(:,2).*cang(:,3)];
end

function dcm = q2dcm( q )
    %   The direction cosine matrix performs the coordinate
    %   transformation of a vector in inertial axes to a vector in body axes.

    qin = q; % don't need to normalize because it is already done
    %qin = quatnormalize( q );

    dcm = zeros(3,3);

    dcm(1,1) = qin(1).^2 + qin(2).^2 - qin(3).^2 - qin(4).^2;
    dcm(1,2) = 2.*(qin(2).*qin(3) + qin(1).*qin(4));
    dcm(1,3) = 2.*(qin(2).*qin(4) - qin(1).*qin(3));
    dcm(2,1) = 2.*(qin(2).*qin(3) - qin(1).*qin(4));
    dcm(2,2) = qin(1).^2 - qin(2).^2 + qin(3).^2 - qin(4).^2;
    dcm(2,3) = 2.*(qin(3).*qin(4) + qin(1).*qin(2));
    dcm(3,1) = 2.*(qin(2).*qin(4) + qin(1).*qin(3));
    dcm(3,2) = 2.*(qin(3).*qin(4) - qin(1).*qin(2));
    dcm(3,3) = qin(1).^2 - qin(2).^2 - qin(3).^2 + qin(4).^2;
end



% function Cd=disrw(F,G,Ts,Rwpsd)
% %----------------------------------------------------------------
% %   function [Cd]=disrw(F,G,T,Rwpsd)
% %
% %   disrw computes the discrete equivalent of continous noise for the
% %   dynamic system described by
% %
% %                            x_dot = Fx + Gw
% %
% %   w is the driving noise.  Ts is the sampling time and Rwpsd
% %   is the power spectral density of the driving noise.
% %
% %---------------------------------------------------------------------
% 
% ZF=zeros(size(F));
% [n,m]=size(G);
% ME=[-F G*Rwpsd*G';
%     ZF F'];
% phi=expm(ME*Ts);
% phi12=phi(1:n,n+1:2*n);
% phi22=phi(n+1:2*n,n+1:2*n);
% Cd=phi22'*phi12;
% 
% end

== matlab function Sensor Data/rotate sensors, normalize magnetometers ==
  data: gyro input inherited; gyro_out output inherited; accel input inherited; mag input inherited; accel_out output inherited; mag_out output inherited; mag_out_norm output inherited
function [gyro_out,accel_out,mag_out,mag_out_norm] = fcn(gyro,accel,mag)
% This block supports an embeddable subset of the MATLAB language.
% See the help menu for details. 

gyro_out     =  [  -gyro(2);  -gyro(1);  -gyro(3)];
accel_out    = -[ -accel(2); -accel(1); -accel(3)];
mag_out      =  [   -mag(2);   -mag(1);   -mag(3)];
mag_out_norm =  mag_out*0.002052459997419;  % mag_out*100/48722.0214405

== matlab function Position-Attitude Filter/Position Filter/Embedded MATLAB Function ==
  data: LLH input inherited; gps_good output inherited; gps_dt_out output inherited
function [gps_good,gps_dt_out] = fcn(LLH)
% This block supports an embeddable subset of the MATLAB language.
% See the help menu for details. 

persistent LL_old
persistent t
persistent gps_dt

if isempty(LL_old)
    t=single(0);
    LL_old=single([0;0]);
    gps_dt = single(10);
end
gps_good=single(0);
t=t+.01;
if LLH(1)-LL_old(1)~=0 ||LLH(2)-LL_old(2)~=0
    gps_dt = t;
    gps_good=single(1);
    LL_old=LLH(1:2);
    t=single(0);
end
gps_dt_out=gps_dt;

== matlab function Position-Attitude Filter/Position Filter/myMux Fun1 ==
  data: u1 input inherited; y output inherited; u2 input inherited; u3 input inherited
function y = myMux3(u1, u2, u3)
% This block supports an embeddable subset of the MATLAB language.
% See the help menu for details. 

y = [u1(1); u2(1); u3(1)];

== matlab function myMux Fun2 ==
  data: u1 input inherited; y output inherited; u2 input inherited
function y = myMux(u1, u2)
% This block supports an embeddable subset of the MATLAB language.
% See the help menu for details. 

y = [u1(1:3); u2(1:3)];

== matlab function Control Surface Input/myMux Fun5 ==
  data: u1 input inherited; y output inherited; u2 input inherited; u3 input inherited; u4 input inherited; u5 input inherited
function y = myMux(u1, u2, u3, u4, u5)
% This block supports an embeddable subset of the MATLAB language.
% See the help menu for details. 

y = [u1(1); u2(1); u3(1); u4(1); u5(1)];

== matlab function Sensor Data/Sensor Suite/If no HIL then Read all the Sensors/myMux Fun4 ==
  data: u1 input inherited; y output inherited; u2 input inherited; u3 input inherited; u4 input inherited; u5 input inherited; u6 input inherited; u7 input inherited; u8 input inherited; u9 input inherited; u10 input inherited; u11 input inherited; u12 input inherited; u13 input inherited
function y = sensMux(u1, u2,u3,u4,u5,u6,u7,u8, u9, u10, u11, u12, u13)
% This block supports an embeddable subset of the MATLAB language.
% See the help menu for details. 

y = [u1(1); u2(1); u3(1); u4(1); u5(1); u6(1); u7(1); u8(1); u9(1); u10(1); u11(1); u12(1); u13(1)];

== matlab function Sensor Data/Sensor Suite/If no HIL then Read all the Sensors/myMux Fun ==
  data: u1 input inherited; y output inherited; u2 input inherited; u3 input inherited; u4 input inherited
function y = myMux(u1, u2, u3, u4)
% This block supports an embeddable subset of the MATLAB language.
% See the help menu for details. 

y = [u1(1); u2(1); u3(1); u4(1)];
